simulink model "sosanh_velocity"  (R2016b)
settings: Solver=VariableStepAuto  StartTime=0.0  StopTime=20  RelTol=1e-3
undefined symbols (not defined in the file): sigbuilder_block
libraries: simulink x1
settings Model: Creator=nguyenquoctruong  LastModifiedBy=nguyenquoctruong

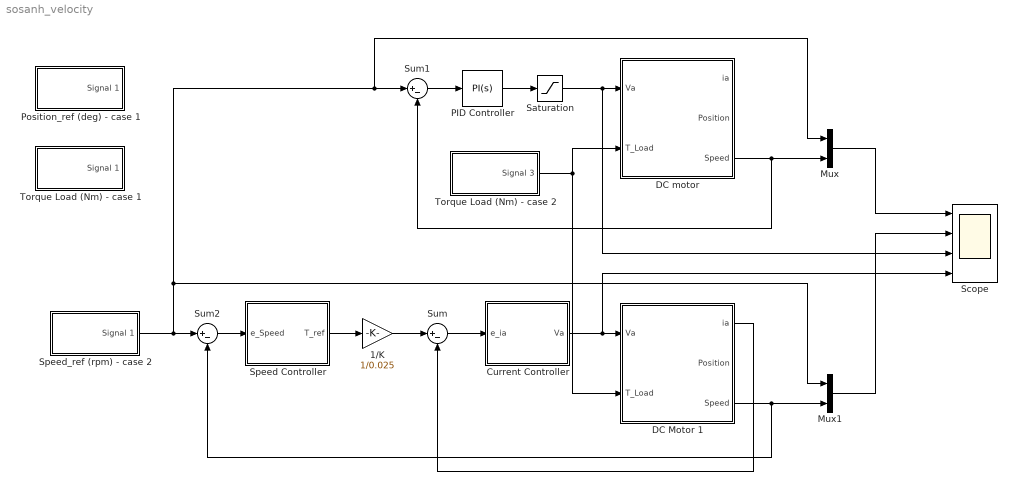
== system sosanh_velocity ==
  1/K : Gain  Gain=1/0.025
  Current Controller : Subsystem  mask{Kp=5, Ki=1, Vmax=12}
      mask prompts: Vmax "Vmax(V)"
  DC Motor 1 : Subsystem  mask{Ra=0.1, K=0.025, Ja=0.0025, La=2*(10^-3), b=0.0002}
      mask prompts: Ra "Ra(Ohm)"; K "K(Vs)"; Ja "Ja(kgm^2)"; La "La(H)"; b "b(Nm.s.rad^-1)"
  "DC motor " : Subsystem  mask{Ra=0.1, K=0.025, Ja=0.002, La=2*(10^-3), b=0.0002}
      mask prompts: Ra "Ra(Ohm)"; K "K(Vs)"; Ja "Ja(kgm^2)"; La "La(H)"; b "b(Nm.s.rad^-1)"
  Mux : Mux  Inputs=2
  Mux1 : Mux  Inputs=2
  PID Controller : simulink/Continuous/PID Controller  Controller=PI  TimeDomain=Continuous-time  SampleTime=-1  IntegratorMethod=Forward Euler  FilterMethod=Forward Euler  Form=Parallel  UseFilter=on  ControllerParametersSource=internal  P=0.1  I=0.09  D=0  N=100  InitialConditionSource=internal  InitialConditionForIntegrator=0  InitialConditionForFilter=0  ExternalReset=none  LimitOutput=off  UpperSaturationLimit=inf  LowerSaturationLimit=-inf  LinearizeAsGain=on  AntiWindupMode=none  Kb=1  TrackingMode=off  Kt=1  PParamMin=[]  PParamMax=[]  IParamMin=[]  IParamMax=[]  DParamMin=[]  DParamMax=[]  NParamMin=[]  NParamMax=[]  KbParamMin=[]  KbParamMax=[]  KtParamMin=[]  KtParamMax=[]  POutMin=[]  POutMax=[]  IOutMin=[]  IOutMax=[]  DOutMin=[]  DOutMax=[]  NOutMin=[]  NOutMax=[]  KbOutMin=[]  KbOutMax=[]  KtOutMin=[]  KtOutMax=[]  IntegratorOutMin=[]  IntegratorOutMax=[]  FilterOutMin=[]  FilterOutMax=[]  SumOutMin=[]  SumOutMax=[]  SumI1OutMin=[]  SumI1OutMax=[]  SumI2OutMin=[]  SumI2OutMax=[]  SumI3OutMin=[]  SumI3OutMax=[]  SumDOutMin=[]  SumDOutMax=[]  SaturationOutMin=[]  SaturationOutMax=[]  IntegratorContinuousStateAttributes=''  IntegratorStateMustResolveToSignalObject=off  IntegratorRTWStateStorageClass=Auto  FilterContinuousStateAttributes=''  FilterStateMustResolveToSignalObject=off  FilterRTWStateStorageClass=Auto  DifferentiatorICPrevScaledInput=0  DifferentiatorOutMin=[]  DifferentiatorOutMax=[]
  Position_ref (deg) - case 1 : Subsystem  Tag=STV Subsys  LoadFcn=sigbuilder_block('load');  StartFcn=sigbuilder_block('start');  StopFcn=sigbuilder_block('stop');  ClipboardFcn=sigbuilder_block('clipboard');  mask(Sigbuilder block){tuvar=[0:10]}
      mask help: Simulink:masks:SigbuilderBlock_MD
      mask init:
      | if ~strcmp(get_param(bdroot(gcbh),'SimulationStatus'),'stopped') tuvar = sigbuilder_block('maskInit'); end
      settings: CopyFcn=sigbuilder_block('copy');  DeleteFcn=sigbuilder_block('delete');  ModelCloseFcn=sigbuilder_block('modelClose');  PreSaveFcn=sigbuilder_block('preSave');  PauseFcn=sigbuilder_block('pause');  ContinueFcn=sigbuilder_block('continue');  NameChangeFcn=sigbuilder_block('namechange');  OpenFcn=sigbuilder_block('open',[196.5 100.5 550.5 359.25 ]);  CloseFcn=sigbuilder_block('close');
      mask Display: plot(0, 0, 100, 100,[2, 2, 32, 32, 2], [68, 8, 8, 68, 68],[32, 2], [38, 38], [32, 19, 2],[53, 60, 44], [32, 17, 17, 2],[16, 16, 31, 31]);txt = getActiveGroup(gcbh);text(2, 100, txt,'verticalAlignment', 'top');
  Saturation : Saturate  UpperLimit=12  LowerLimit=-12
  Scope : Scope  NumInputPorts=4
  Speed Controller : Subsystem  mask{Kp=3, Ki=0.01, Tmax=2.66}
      mask prompts: Tmax "Tmax(Nm)"
  Speed_ref (rpm) - case 2 : Subsystem  Tag=STV Subsys  LoadFcn=sigbuilder_block('load');  StartFcn=sigbuilder_block('start');  StopFcn=sigbuilder_block('stop');  ClipboardFcn=sigbuilder_block('clipboard');  mask(Sigbuilder block){tuvar=[0:10]}
      mask help: Simulink:masks:SigbuilderBlock_MD
      mask init:
      | if ~strcmp(get_param(bdroot(gcbh),'SimulationStatus'),'stopped') tuvar = sigbuilder_block('maskInit'); end
      settings: CopyFcn=sigbuilder_block('copy');  DeleteFcn=sigbuilder_block('delete');  ModelCloseFcn=sigbuilder_block('modelClose');  PreSaveFcn=sigbuilder_block('preSave');  PauseFcn=sigbuilder_block('pause');  ContinueFcn=sigbuilder_block('continue');  NameChangeFcn=sigbuilder_block('namechange');  OpenFcn=sigbuilder_block('open',[115.5 51 550.5 359.25 ]);  CloseFcn=sigbuilder_block('close');
      mask Display: plot(0, 0, 100, 100,[2, 2, 32, 32, 2], [68, 8, 8, 68, 68],[32, 2], [38, 38], [32, 19, 2],[53, 60, 44], [32, 17, 17, 2],[16, 16, 31, 31]);txt = getActiveGroup(gcbh);text(2, 100, txt,'verticalAlignment', 'top');
  Sum : Sum  Inputs=|+-
  Sum1 : Sum  Inputs=|+-
  Sum2 : Sum  Inputs=|+-
  Torque Load (Nm) - case 1 : Subsystem  Tag=STV Subsys  LoadFcn=sigbuilder_block('load');  StartFcn=sigbuilder_block('start');  StopFcn=sigbuilder_block('stop');  ClipboardFcn=sigbuilder_block('clipboard');  mask(Sigbuilder block){tuvar=[0:10]}
      mask help: Simulink:masks:SigbuilderBlock_MD
      mask init:
      | if ~strcmp(get_param(bdroot(gcbh),'SimulationStatus'),'stopped') tuvar = sigbuilder_block('maskInit'); end
      settings: CopyFcn=sigbuilder_block('copy');  DeleteFcn=sigbuilder_block('delete');  ModelCloseFcn=sigbuilder_block('modelClose');  PreSaveFcn=sigbuilder_block('preSave');  PauseFcn=sigbuilder_block('pause');  ContinueFcn=sigbuilder_block('continue');  NameChangeFcn=sigbuilder_block('namechange');  OpenFcn=sigbuilder_block('open',[196.5 100.5 550.5 359.25 ]);  CloseFcn=sigbuilder_block('close');
      mask Display: plot(0, 0, 100, 100,[2, 2, 32, 32, 2], [68, 8, 8, 68, 68],[32, 2], [38, 38], [32, 19, 2],[53, 60, 44], [32, 17, 17, 2],[16, 16, 31, 31]);txt = getActiveGroup(gcbh);text(2, 100, txt,'verticalAlignment', 'top');
  Torque Load (Nm) - case 2 : Subsystem  Tag=STV Subsys  LoadFcn=sigbuilder_block('load');  StartFcn=sigbuilder_block('start');  StopFcn=sigbuilder_block('stop');  ClipboardFcn=sigbuilder_block('clipboard');  mask(Sigbuilder block){tuvar=[0:10]}
      mask help: Simulink:masks:SigbuilderBlock_MD
      mask init:
      | if ~strcmp(get_param(bdroot(gcbh),'SimulationStatus'),'stopped') tuvar = sigbuilder_block('maskInit'); end
      settings: CopyFcn=sigbuilder_block('copy');  DeleteFcn=sigbuilder_block('delete');  ModelCloseFcn=sigbuilder_block('modelClose');  PreSaveFcn=sigbuilder_block('preSave');  PauseFcn=sigbuilder_block('pause');  ContinueFcn=sigbuilder_block('continue');  NameChangeFcn=sigbuilder_block('namechange');  OpenFcn=sigbuilder_block('open',[196.5 100.5 550.5 359.25 ]);  CloseFcn=sigbuilder_block('close');
      mask Display: plot(0, 0, 100, 100,[2, 2, 32, 32, 2], [68, 8, 8, 68, 68],[32, 2], [38, 38], [32, 19, 2],[53, 60, 44], [32, 17, 17, 2],[16, 16, 31, 31]);txt = getActiveGroup(gcbh);text(2, 100, txt,'verticalAlignment', 'top');
  wires:
  PID Controller/1 -> Saturation/1
  Sum1/1 -> PID Controller/1
  Saturation/1 -> Scope/3, "DC motor "/1("Va ")
  DC Motor 1/1(ia) -> Sum/2
  Sum2/1 -> Speed Controller/1(e_Speed)
  1/K/1 -> Sum/1
  Current Controller/1("Va ") -> Scope/4, DC Motor 1/1("Va ")
  Sum/1 -> Current Controller/1(e_ia)
  Speed Controller/1("T_ref ") -> 1/K/1
  Mux1/1 -> Scope/2
  Mux/1 -> Scope/1
  Torque Load (Nm) - case 2/1(Signal 3) -> "DC motor "/2(T_Load), DC Motor 1/2(T_Load)
  Speed_ref (rpm) - case 2/1(Signal 1) -> Sum2/1, Mux1/1, Mux/1, Sum1/1
  "DC motor "/3("Speed ") -> Mux/2, Sum1/2
  DC Motor 1/3("Speed ") -> Mux1/2, Sum2/2

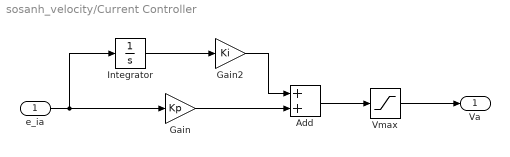
== system sosanh_velocity/Current Controller ==
  e_ia : Inport
  Add : Sum
  Gain : Gain  Gain=Kp
  Gain2 : Gain  Gain=Ki
  Integrator : Integrator
  Vmax : Saturate  UpperLimit=Vmax  LowerLimit=-Vmax
  "Va " : Outport
  wires:
  Integrator/1 -> Gain2/1
  e_ia/1 -> Integrator/1, Gain/1
  Gain2/1 -> Add/1
  Add/1 -> Vmax/1
  Vmax/1 -> "Va "/1
  Gain/1 -> Add/2

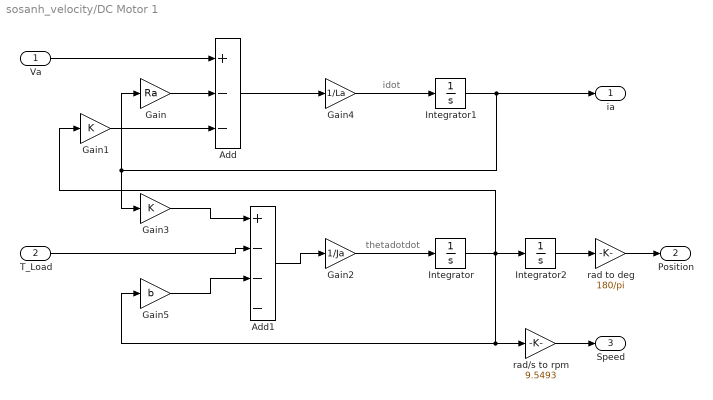
== system sosanh_velocity/DC Motor 1 ==
  note: thetadotdot
  note: idot
  "Va " : Inport
  T_Load : Inport  Port=2
  Add : Sum  Inputs=+--
  Add1 : Sum  Inputs=+---
  Gain : Gain  Gain=Ra
  Gain1 : Gain  Gain=K
  Gain2 : Gain  Gain=1/Ja
  Gain3 : Gain  Gain=K
  Gain4 : Gain  Gain=1/La
  Gain5 : Gain  Gain=b
  Integrator : Integrator
  Integrator1 : Integrator
  Integrator2 : Integrator
  rad to deg : Gain  Gain=180/pi
  rad/s to rpm : Gain  Gain=9.5493
  ia : Outport
  Position : Outport  Port=2
  "Speed " : Outport  Port=3
  wires:
  Gain/1 -> Add/2
  T_Load/1 -> Add1/2
  Gain1/1 -> Add/3
  Gain3/1 -> Add1/1
  "Va "/1 -> Add/1
  Gain4/1 -> Integrator1/1
  Add/1 -> Gain4/1
  Add1/1 -> Gain2/1
  Gain2/1 -> Integrator/1
  Integrator1/1 -> ia/1, Gain/1, Gain3/1
  Integrator/1 -> Gain1/1, Integrator2/1, Gain5/1, rad/s to rpm/1
  Gain5/1 -> Add1/3
  rad/s to rpm/1 -> "Speed "/1
  Integrator2/1 -> rad to deg/1
  rad to deg/1 -> Position/1

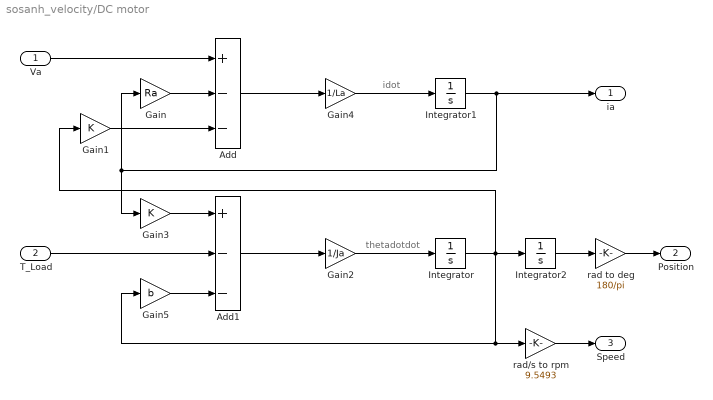
== system sosanh_velocity/DC motor  ==
  note: thetadotdot
  note: idot
  "Va " : Inport
  T_Load : Inport  Port=2
  Add : Sum  Inputs=+--
  Add1 : Sum  Inputs=+--
  Gain : Gain  Gain=Ra
  Gain1 : Gain  Gain=K
  Gain2 : Gain  Gain=1/Ja
  Gain3 : Gain  Gain=K
  Gain4 : Gain  Gain=1/La
  Gain5 : Gain  Gain=b
  Integrator : Integrator
  Integrator1 : Integrator
  Integrator2 : Integrator
  rad to deg : Gain  Gain=180/pi
  rad/s to rpm : Gain  Gain=9.5493
  ia : Outport
  Position : Outport  Port=2
  "Speed " : Outport  Port=3
  wires:
  Gain/1 -> Add/2
  T_Load/1 -> Add1/2
  Gain1/1 -> Add/3
  Gain3/1 -> Add1/1
  "Va "/1 -> Add/1
  Gain4/1 -> Integrator1/1
  Add/1 -> Gain4/1
  Add1/1 -> Gain2/1
  Gain2/1 -> Integrator/1
  Integrator1/1 -> ia/1, Gain/1, Gain3/1
  Integrator/1 -> Gain1/1, Integrator2/1, Gain5/1, rad/s to rpm/1
  Gain5/1 -> Add1/3
  rad/s to rpm/1 -> "Speed "/1
  Integrator2/1 -> rad to deg/1
  rad to deg/1 -> Position/1

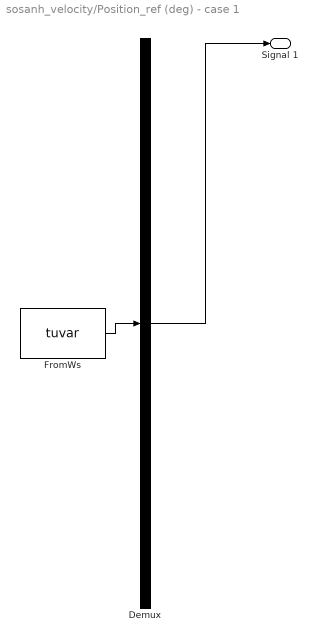
== system sosanh_velocity/Position_ref (deg) - case 1 ==
  Demux : Demux  Tag=STV Demux  Outputs=1
  FromWs : FromWorkspace  Tag=STV FromWs  VariableName=tuvar  SampleTime=0
      SigBuilderData=|
      | common.afterFinalStr = 'Extrapolate'
      | common.sampleTime = 0
      | dataSet.timeRange = [0 20]
      | dataSet.name = 'Group 1'
      | sbobj.Groups.Name = 'Group 1'
      | sbobj.Groups.Signals.Name = 'Signal 1'
      | sbobj.Groups.Signals.XData = [0 2.2 2.2 10.4 10.4 20]
      | sbobj.Groups.Signals.YData = [0 0 60 60 360 360]
      | sbobj.Groups.TimeRange = [0 20]
  Signal 1 : Outport  Tag=STV Outport
  wires:
  Demux/1 -> Signal 1/1
  FromWs/1 -> Demux/1

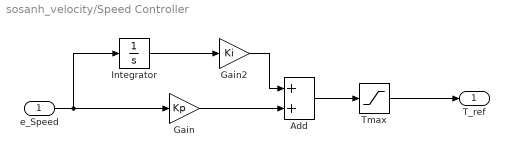
== system sosanh_velocity/Speed Controller ==
  e_Speed : Inport
  Add : Sum
  Gain : Gain  Gain=Kp
  Gain2 : Gain  Gain=Ki
  Integrator : Integrator
  Tmax : Saturate  UpperLimit=Tmax  LowerLimit=-Tmax
  "T_ref " : Outport
  wires:
  Tmax/1 -> "T_ref "/1
  Add/1 -> Tmax/1
  Gain2/1 -> Add/1
  Gain/1 -> Add/2
  e_Speed/1 -> Gain/1, Integrator/1
  Integrator/1 -> Gain2/1

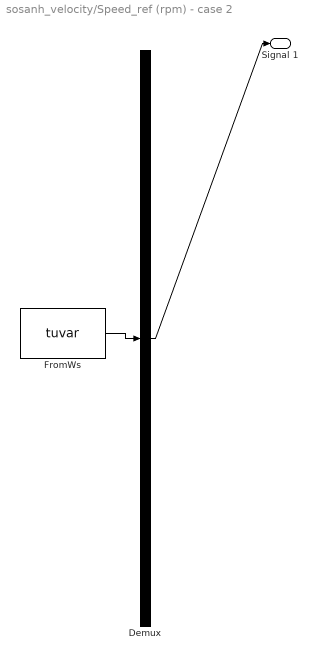
== system sosanh_velocity/Speed_ref (rpm) - case 2 ==
  Demux : Demux  Tag=STV Demux  Outputs=1
  FromWs : FromWorkspace  Tag=STV FromWs  VariableName=tuvar  SampleTime=0
      SigBuilderData=|
      | common.afterFinalStr = 'Extrapolate'
      | common.sampleTime = 0
      | dataSet.timeRange = [0 20]
      | dataSet.name = 'Group 1'
      | sbobj.Groups.Name = 'Group 1'
      | sbobj.Groups.Signals.Name = 'Signal 1'
      | sbobj.Groups.Signals.XData = [0 1 1 2 3 3 4 4 5 5 6 6 7 7 8 8 9 9 10 10 11 11 12 13 14 14 15 15 16 16 17 17 18 18 19 20]
      | sbobj.Groups.Signals.YData = [0 0 2760 2760 2760 1700 1700 2580 2580 2180 2180 2420 2420 2840 2840 1500 1500 1880 1880 2480 2480 3500 3500 3500 3500 3000 3000 3160 3160 2820 2820 2080 2080 1350 1350 1350]
      | sbobj.Groups.TimeRange = [0 20]
  Signal 1 : Outport  Tag=STV Outport
  wires:
  FromWs/1 -> Demux/1
  Demux/1 -> Signal 1/1

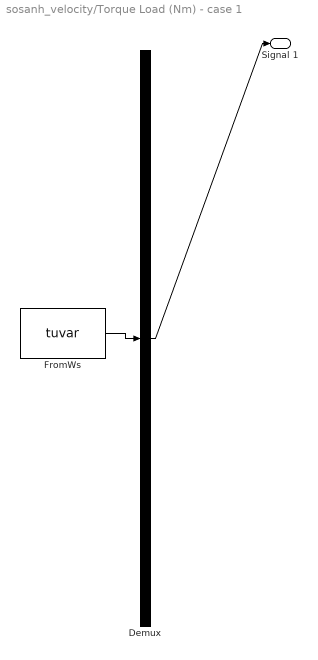
== system sosanh_velocity/Torque Load (Nm) - case 1 ==
  Demux : Demux  Tag=STV Demux  Outputs=1
  FromWs : FromWorkspace  Tag=STV FromWs  VariableName=tuvar  SampleTime=0
      SigBuilderData=|
      | common.afterFinalStr = 'Extrapolate'
      | common.sampleTime = 0
      | dataSet.timeRange = [5 15]
      | dataSet.name = 'Group 1'
      | sbobj.Groups.Name = 'Group 1'
      | sbobj.Groups.Signals.Name = 'Signal 1'
      | sbobj.Groups.Signals.XData = [5 5.2 5.3 5.3 5.5 5.5 5.7 5.7 6 6 6.1 6.1 6.3 6.3 6.4 6.4 6.5 6.5 6.7 6.7 7.1 7.1 7.2 7.2 7.7 7.7 7.8 7.8 7.9 7.9 8 8 8.1 8.1 8.5 8.5 8.7 8.7 8.8 8.8 8.9 8.9 9.2 9.2 9.4 9.4 9.7 9.7 10 10 10.1 10.1 10.3 10.3 10.6 10.6 10.7 10.7 10.8 10.8 10.9 10.9 11 11 11.1 11.1 11.2 11.2 11.7 11.7 12 12 12.1 12.1 12.2 12.2 12.3 12.3 12.4 12.4 12.5 12.5 12.8 12.8 12.9 12.9 13.1 13.1 13.5 13.5 13.6 13.6 13.8 13.8 13.9 13.9 14 14 14.2 14.2 14.5 14.5 14.6 14.6 14.7 14.7 15]
      | sbobj.Groups.Signals.YData = [0 0 0 1 1 0 0 1 1 0 0 1 1 0 0 1 1 0 0 1 1 0 0 1 1 0 0 1 1 0 0 1 1 0 0 1 1 0 0 1 1 0 0 1 1 0 0 1 1 0 0 1 1 0 0 1 1 0 0 1 1 0 0 1 1 0 0 1 1 0 0 1 1 0 0 1 1 0 0 1 1 0 0 1 1 0 0 1 1 0 0 1 1 0 0 1 1 0 0 1 1 0 0 1 1 0 0]
      | sbobj.Groups.TimeRange = [5 15]
  Signal 1 : Outport  Tag=STV Outport
  wires:
  FromWs/1 -> Demux/1
  Demux/1 -> Signal 1/1

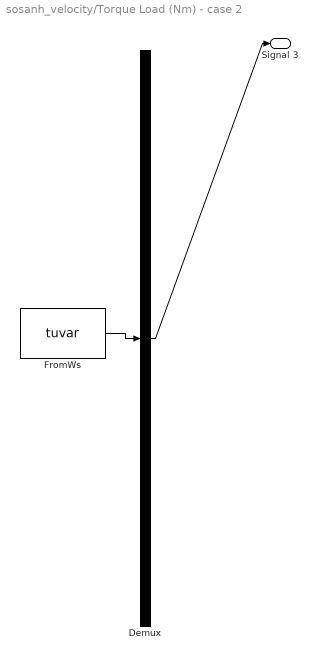
== system sosanh_velocity/Torque Load (Nm) - case 2 ==
  Demux : Demux  Tag=STV Demux  Outputs=1
  FromWs : FromWorkspace  Tag=STV FromWs  VariableName=tuvar  SampleTime=0
      SigBuilderData=|
      | common.afterFinalStr = 'Extrapolate'
      | common.sampleTime = 0
      | dataSet.timeRange = [0 20]
      | dataSet.name = 'Group 1'
      | sbobj.Groups.Name = 'Group 1'
      | sbobj.Groups.Signals.Name = 'Signal 3'
      | sbobj.Groups.Signals.XData = [0 1 1 4.6 4.6 12.5 12.5 20]
      | sbobj.Groups.Signals.YData = [0 0 1 1 0.5 0.5 0.355 0.355]
      | sbobj.Groups.TimeRange = [0 20]
  Signal 3 : Outport  Tag=STV Outport
  wires:
  FromWs/1 -> Demux/1
  Demux/1 -> Signal 3/1
